simulink model "test_GRM_Airframe"  (R2019b)
settings: Solver=FixedStepAuto  StartTime=0.0  StopTime=60  FixedStep=0.001  RelTol=1e-3
PreLoadFcn:
  | addpath('init_functions');
  | init_grm;
  | addpath('parameters');
  | para_def_grm;
values from neighbouring files (symbols this model uses):
  a_vBEW = 0    [init_grm.m]
  act_dmp = 0.6322    [para_def_grm.m]
  act_omega = 59.9250    (= 59.925)    [para_def_grm.m]
  aero = load('aero.mat')    [para_def_grm.m]
  c_be = -6.5e-3    (= -0.0065)    [init_grm.m]
  c_h_geop0 = 0    [init_grm.m]
  c_h_geope = 11e3    (= 11000)    [init_grm.m]
  c_pa0 = 101325    [init_grm.m]
  c_pe = -c_g0/c_be/sgc    (= 5.25587981272)    [init_grm.m]
  c_r0 = 6371000.79    [init_grm.m]
  c_rot = 7.292115e-5    (= 7.292115e-05)    [init_grm.m]
  c_Tmp0 = 288.15    [init_grm.m]
  chW = pi/2    (= 1.57079632679)    [init_grm.m]
  D = JD - 2451545.0    [init_grm.m]
  d_siB_0 = 0    [para_def_grm.m]
  d_siB_max = deg2rad(1200)    [para_def_grm.m]
  d_siB_min = deg2rad(-1200)    [para_def_grm.m]
  dd_siB_max = deg2rad(50000)    [para_def_grm.m]
  dd_siB_min = deg2rad(-50000)    [para_def_grm.m]
  de_JBBB_xx = JBBB_xx_0 - JBBB_xx_e    (= 0)    [para_def_grm.m]
  de_JBBB_yy = JBBB_yy_0 - JBBB_yy_e    (= 0)    [para_def_grm.m]
  de_JBBB_zz = JBBB_zz_0 - JBBB_zz_e    (= 0)    [para_def_grm.m]
  de_mM = m_fuel_lookup(end)    [para_def_grm.m]
  e_pa = 0    [init_grm.m]
  e_Tmp = 0    [init_grm.m]
  F_prp = [450.52;428.7;423.25;391.61;352.34;304.35;266.17;243.26;216.92 ... (first row only)    [para_def_grm.m]
  flag_I_aero_switch = 1    [init_grm.m]
  flag_I_flat = 1    [init_grm.m]
  flag_I_gravity_switch = 1    [init_grm.m]
  flag_I_rot = 0    [init_grm.m]
  hcr = 1.4    [init_grm.m]
  J0PB_e = TBP*J0PP_e*TBP'    [para_def_grm.m]
  JMMM_0 = TBP*J0PP_0*TBP'    [para_def_grm.m]
  JMMM_e = TBP*J0PP_e*TBP'    [para_def_grm.m]
  lat_0 = 0    [init_grm.m]
  lon_0 = 0    [init_grm.m]
  m0 = mB_0    (= 3.30977)    [para_def_grm.m]
  m_fuel_lookup = [0;0.0573;0.1127;0.1667;0.2186;0.2681;0.3149;0.3588 ... (first row only)    [para_def_grm.m]
  mB_0 = 3.30977    [para_def_grm.m]
  mM_0 = 1.119    [para_def_grm.m]
  mM_e = de_mM    [para_def_grm.m]
  p0PB = [x0PB;y0PB;z0PB]    [para_def_grm.m]
  pBII_0 = TIE_0*pBEE_0    [init_grm.m]
  pMPB = [xMPB;yMPB;zMPB]    [para_def_grm.m]
  pNPB = [0;0;0]    [para_def_grm.m]
  qEG_0 = q12_from_T12(TEG)    [init_grm.m]
  qIB_0 = qumul(qIG_0,qGB_0)    [init_grm.m]
  qIE_0 = q12_from_T12(TIE_0)    [init_grm.m]
  sgc = 287.05287    [init_grm.m]
  siB_0 = 0    [para_def_grm.m]
  siB_max = deg2rad(30)    [para_def_grm.m]
  siB_min = deg2rad(-30)    [para_def_grm.m]
  t_prp1 = [0.04;0.28;0.54;1;1.48;1.99;2.51;3;3.5;3.67;3.82;4]    [para_def_grm.m]
  t_prp2 = t_prp2'    [para_def_grm.m]
  T_sim_lnch = -5    [init_grm.m]
  Tr3r4 = [1,1,1,1;1,1,-1,-1;-1,1,1,-1]*0.25    [para_def_grm.m]
  Tr4r3 = [1,1,-1;1,1,1;1,-1,1;1,-1,-1]    [para_def_grm.m]
  tRRR = 0    [para_def_grm.m]
  unc_a_vBEW_bl = 0    [para_def_grm.m]
  unc_act_bl = 0    [para_def_grm.m]
  unc_act_off = 0    [para_def_grm.m]
  unc_act_scale = 1    [para_def_grm.m]
  unc_aero_Cl_scale = 1    [para_def_grm.m]
  unc_aero_Cm_scale = 1    [para_def_grm.m]
  unc_aero_Cn_scale = 1    [para_def_grm.m]
  unc_aero_Cx_scale = 1    [para_def_grm.m]
  unc_aero_Cy_scale = 1    [para_def_grm.m]
  unc_aero_Cz_scale = 1    [para_def_grm.m]
  unc_cg_x = 0    [para_def_grm.m]
  unc_cg_y = 0    [para_def_grm.m]
  unc_cg_z = 0    [para_def_grm.m]
  unc_chW_bl = 0    [para_def_grm.m]
  unc_fin_def_pitch = 0    [para_def_grm.m]
  unc_fin_def_roll = 0    [para_def_grm.m]
  unc_fin_def_yaw = 0    [para_def_grm.m]
  unc_mB_bl = 0    [para_def_grm.m]
  unc_mB_scale = 1    [para_def_grm.m]
  unc_moi_Jxx = 0    [para_def_grm.m]
  unc_moi_Jyy = 0    [para_def_grm.m]
  unc_moi_Jzz = 0    [para_def_grm.m]
  unc_prp_scale = 1    [para_def_grm.m]
  unc_prp_x = 0    [para_def_grm.m]
  unc_prp_y = 0    [para_def_grm.m]
  unc_prp_z = 0    [para_def_grm.m]
  vBII_0 = vBEE_0 + cross(wIEI_0,pBII_0)    [init_grm.m]
  wBIB_0 = r2_from_r1_trans_q21(wBII_0,qBI_0)    [init_grm.m]
  x0PB = -0.5    [para_def_grm.m]
  xMPB = -0.9    [para_def_grm.m]
  y0PB = 0    [para_def_grm.m]
  yMPB = 0    [para_def_grm.m]
  z0PB = 0    [para_def_grm.m]
  zMPB = 0    [para_def_grm.m]
undefined symbols (not defined in the file or in its folder): c_b_WGS, c_flat, c_grav, c_rsma, d_mB_lookup, t_dmB
libraries: simulink_extras x14, simulink x3
(part 3 of 6)

== system test_GRM_Airframe/GRM_Airframe/rb_eom/calc_bus_flight_dyn_bus_entries/Subsystem2 ==
  TIE : Inport
  pBII : Inport  Port=2
  Constant : Constant  Value=lon_0
  Constant1 : Constant  Value=flag_I_flat
  Constant2 : Constant  Value=lat_0
  Demux : Demux  Outputs=3
  Demux1 : Demux  Outputs=3
  Gain : Gain  Gain=-1
  Math Function : Math  Operator=transpose  SaturateOnIntegerOverflow=on
  Product : Product  Multiplication=Matrix(*)
  Switch : Switch  Criteria=u2 > Threshold
  Terminator : Terminator
  Terminator1 : Terminator
  Vector Concatenate : Concatenate  NumInputs=3
  Vector Concatenate1 : Concatenate  NumInputs=3
  trafo_E_to_geodetic : Subsystem  mask(Transformation der ECEF Position in geodätische Größen){}
      mask help: Dieser Block transformiert die Position im ECEF KOS in die geodätische Länge, Breite und Höhe
      mask init:
      | [c_mue, c_rsma, c_flat] = init_transformations_earth;
      mask Help:
      | Name:
      | 
      |     trafo_E_to_geodetic
      | 
      | Beschreibung:
      | 
      |     Dieser Block transformiert die Position im ECEF KOS in die geodätische
      |     Länge, Breite und Höhe.
      | 
      | Inputs   [size]  [data type] [unit]:
      | 
      |     pBEE    [3] [double] [m]
      | 
      | Outputs  [size]  [data type] [unit]:
      | 
      |     long  [1] [double] [rad]
      |     lat   [1] [double] [rad]
      |     alt   [1] [double] [m]
      | 
      | Parameter
      | 
      |    c_rsma
      |    c_flat
  lon : Outport  VectorParamsAs1DForOutWhenUnconnected=off
  lat : Outport  Port=2  VectorParamsAs1DForOutWhenUnconnected=off
  hBE : Outport  Port=3  VectorParamsAs1DForOutWhenUnconnected=off
  wires:
  Demux1/2 -> lat/1  "lat"
  pBII/1 -> Demux/1, Product/2
  Product/1 -> trafo_E_to_geodetic/1(pBEE)  "pBEE"
  Demux1/1 -> lon/1  "lon"
  Demux1/3 -> hBE/1  "hBE"
  trafo_E_to_geodetic/1(lon) -> Vector Concatenate/1  "lon"
  trafo_E_to_geodetic/2(lat) -> Vector Concatenate/2  "lat"
  trafo_E_to_geodetic/3(alt) -> Vector Concatenate/3  "alt"
  Demux/1 -> Terminator/1
  Demux/2 -> Terminator1/1
  Demux/3 -> Gain/1
  Gain/1 -> Vector Concatenate1/3
  Constant/1 -> Vector Concatenate1/1
  Constant2/1 -> Vector Concatenate1/2
  Vector Concatenate/1 -> Switch/3
  Constant1/1 -> Switch/2
  Vector Concatenate1/1 -> Switch/1
  Switch/1 -> Demux1/1
  TIE/1 -> Math Function/1
  Math Function/1 -> Product/1  "TEI"

== system test_GRM_Airframe/GRM_Airframe/rb_eom/calc_bus_flight_dyn_bus_entries/quaternion_to_euler_angles ==
  note: Inputs [size]:
      |
      | quaternion [4]
  note: Outputs [size]:
      |
      | roll angle [1]
      | pitch angle [1]
      | yaw angle [1]
  note: Um numerische Probleme zu
      | vermeiden, wird hier eine Saturiierung
      | benutzt.
  q : Inport  PortDimensions=4
  Add : Sum
  Add1 : Sum  Inputs=+--
  Add2 : Sum  Inputs=+-
  Add3 : Sum
  Add4 : Sum  Inputs=+--
  Complex to Real-Imag : ComplexToRealImag  Output=Real
  Constant : Constant  Value=0.5
  Constant1 : Constant  Value=0.5
  Demux : Demux
  Gain : Gain  Gain=2
  Product{,1..9} (10 alike) : Product
  Saturation : Saturate  UpperLimit=1  LowerLimit=-1
      settings: AttributesFormatString=|
      | %<UpperLimit>
      | %<LowerLimit>
  Trigonometric Function : Trigonometry  Operator=atan2
  Trigonometric Function1 : Trigonometry  Operator=asin
  Trigonometric Function2 : Trigonometry  Operator=atan2
  Vector Concatenate : Concatenate  NumInputs=3
  eulx : Outport  VectorParamsAs1DForOutWhenUnconnected=off
  wires:
  Saturation/1 -> Trigonometric Function1/1
  Gain/1 -> Saturation/1
  Demux/3 -> Product5/2, Product1/2, Product7/1, Product9/1, Product9/2  "3"
  Constant1/1 -> Add4/1
  Product8/1 -> Add4/2
  Product9/1 -> Add4/3
  Constant/1 -> Add1/1
  Demux/2 -> Product6/2, Product8/1, Product8/2, Product1/1, Product3/1, Product3/2, Product4/1  "2"
  Demux/1 -> Product5/1, Product6/1, Product/1, Product2/1, Product2/2  "1"
  Demux/4 -> Product/2, Product4/2, Product7/2  "4"
  q/1 -> Demux/1
  Add1/1 -> Trigonometric Function/2
  Add2/1 -> Gain/1
  Add4/1 -> Trigonometric Function2/2
  Add3/1 -> Trigonometric Function2/1
  Product6/1 -> Add3/1
  Product7/1 -> Add3/2
  Product4/1 -> Add2/1
  Product5/1 -> Add2/2
  Product2/1 -> Add1/2
  Product3/1 -> Add1/3
  Product/1 -> Add/1
  Product1/1 -> Add/2
  Add/1 -> Trigonometric Function/1
  Trigonometric Function/1 -> Vector Concatenate/1
  Trigonometric Function1/1 -> Vector Concatenate/2
  Trigonometric Function2/1 -> Vector Concatenate/3
  Complex to Real-Imag/1 -> eulx/1
  Vector Concatenate/1 -> Complex to Real-Imag/1

== system test_GRM_Airframe/GRM_Airframe/rb_eom/eom_6dof/Rigid_Body_EOM_6_DOF ==
  FBTX : Inport  PortDimensions=[3,1]
  MBTB : Inport  Port=2  PortDimensions=[3,1]
  mB : Inport  Port=3  PortDimensions=[1]
  x0 : Inport  Port=4
  JBB : Inport  Port=5  PortDimensions=[3,3]
  d_JBB : Inport  Port=6  PortDimensions=[3,3]
  Bus Selector : BusSelector  OutputSignals=qIB,vBII,wBIB
  Constant : Constant  Value=flag_Kraft
  Integration : Subsystem
  Math Function2 : Math  Operator=transpose  SaturateOnIntegerOverflow=on
  Product2 : Product  Multiplication=Matrix(*)
  Switch : Switch  Criteria=u2 > Threshold  Threshold=1
  T12_from_q12 : Subsystem
      mask help: Transforms a quaternion into a Direction Cosine Matrix
      mask Help:
      | Name:
      | 
      |     T12_from_q12
      | 
      | Description:
      | 
      |     This block implements the transformation of a quaternion into the
      |     corresponding direction cosine matrix DCM.
      | 
      | Inputs  [size] [data type] [unit]:
      | 
      |     quaternion q12 [4] [double] [-]
      | 
      | Outputs  [size] [data type] [unit]:
      | 
      |     direction cosine matrix T12  [3x3] [double] [-]
      mask Display:
      | %port_label('input', 1, 'q12')
      | %port_label('output', 1, 'T12')
      | disp('q \rightarrow DCM','texmode','on')
  rb_eom_6dof : Subsystem
  rb_eom : Outport  VectorParamsAs1DForOutWhenUnconnected=off
  wires:
  rb_eom_6dof/4(d_wBIB) -> Integration/4(d_wBIB)  "d_wBIB"
  JBB/1 -> rb_eom_6dof/3(JBB)
  d_JBB/1 -> rb_eom_6dof/5(d_JBB)
  mB/1 -> rb_eom_6dof/2(mB)
  MBTB/1 -> rb_eom_6dof/4(MBTB)
  Switch/1 -> rb_eom_6dof/1(FBTB)
  Constant/1 -> Switch/2
  Product2/1 -> Switch/3
  FBTX/1 -> Product2/2, Switch/1
  Math Function2/1 -> Product2/1
  T12_from_q12/1(T12) -> Math Function2/1
  Bus Selector/2 -> rb_eom_6dof/7(vBII)  "<vBII>"
  x0/1 -> Integration/5(x0)
  Bus Selector/1 -> rb_eom_6dof/6(qIB), T12_from_q12/1(q12)  "<qIB>"
  Bus Selector/3 -> rb_eom_6dof/8(wBIB)  "<wBIB>"
  rb_eom_6dof/1(d_pBII) -> Integration/1(d_pBII)  "d_pBII"
  rb_eom_6dof/2(d_vBII) -> Integration/2(d_vBII)  "d_vBII"
  rb_eom_6dof/3(d_qIB) -> Integration/3(d_qIB)  "d_qIB"
  Integration/1(eom) -> Bus Selector/1, rb_eom/1

== system test_GRM_Airframe/GRM_Airframe/stream_flow/calc_stream_flow/Subsystem1 ==
  vWEB : Inport
  vBEB : Inport  Port=2
  wBIB : Inport  Port=3
  rho : Inport  Port=4
  sos : Inport  Port=5
  AoA_Sideslip_Alphatot_Phi : Subsystem
      mask help:
      | Aus den Komponenten der Geschwindigkeit im ECEF-System, dargestellt im Body-System vBEB
      | werden Anstellwinkel (alpha), Schiebewinkel (beta), totaler Anstellwinkel (alpha_T) sowie Rollwinkel (phi) berechnet.
      | Die Ausgabe erfolgt als Bus in [rad]
      mask Help:
      | Name:
      | 
      |    AoA_sideslip_alphatot_phi
      | 
      | Beschreibung:
      | 
      |   Dieser Block berechnet Anstellwinkel, Schiebewinkel, totalen Anstellwinkel und Rollwinkel in [rad]
      |   aus der Geschwindigkeit vBEB (ECEF-System dargestellt in Body-Koordinaten)
      | 
      | Inputs   [dimension]  [data type] [unit]:
      | 
      |     vBEB    [3] [double] [m/s]
      | 
      | Outputs  [dimension]  [data type] [unit]:
      | 
      | aero_angle_bus [4] [bus] [-]
      |     alpha     [1] [double] [rad]
      |     beta       [1] [double] [rad]
      |     alpha_T [1] [double] [rad]
      |     phi         [1] [double] [rad]
      mask Display:
      | %port_label('input', 1, 'vBEB')
      | %port_label('output', 1, 'aero_angles')
      | disp('vBEB \rightarrow \alpha \beta \alpha_T \phi','texmode','on')
  Bus Selector : BusSelector  OutputSignals=al,be,th,fi
  Constant : Constant  Value=0.5
  Divide : Product  Inputs=*/
  Math Function1 : Math  Operator=square  SaturateOnIntegerOverflow=on
  Product1 : Product  Inputs=3
  Subtract : Sum  Inputs=+-
  calc_nondimensional_rates : Subsystem
  norm_of_vector : Subsystem
      mask help: computes the norm of a vector
      mask Help:
      | Name:
      | 
      |     norm_of_vector
      | 
      | Description:
      | 
      |     This block computes the L2-norm (length) of a vector.
      | 
      | Inputs  [size] [data type] [unit]:
      | 
      |     vector  [3] [double] [-]
      | 
      | Outputs  [size] [data type] [unit]:
      | 
      |     norm of vector  [1] [double] [-]
      mask Display: disp (' norm(r) ')
  al : Outport  VectorParamsAs1DForOutWhenUnconnected=off
  be : Outport  Port=2  VectorParamsAs1DForOutWhenUnconnected=off
  qdynB : Outport  Port=3  VectorParamsAs1DForOutWhenUnconnected=off
  MaB : Outport  Port=4  VectorParamsAs1DForOutWhenUnconnected=off
  a_vB : Outport  Port=5  VectorParamsAs1DForOutWhenUnconnected=off
  wBIB_star : Outport  Port=6  VectorParamsAs1DForOutWhenUnconnected=off
  th : Outport  Port=7  VectorParamsAs1DForOutWhenUnconnected=off
  fi : Outport  Port=8  VectorParamsAs1DForOutWhenUnconnected=off
  wires:
  sos/1 -> Divide/2
  AoA_Sideslip_Alphatot_Phi/1(aero_angles) -> Bus Selector/1
  vBEB/1 -> Subtract/1
  norm_of_vector/1(norm_of_vector) -> Math Function1/1, calc_nondimensional_rates/1(a_vB), a_vB/1, Divide/1  "a_vB"
  Product1/1 -> qdynB/1  "qdynB"
  Math Function1/1 -> Product1/1
  Constant/1 -> Product1/2
  Divide/1 -> MaB/1  "MaB"
  Bus Selector/2 -> be/1  "<be>"
  rho/1 -> Product1/3
  Bus Selector/1 -> al/1  "<al>"
  wBIB/1 -> calc_nondimensional_rates/2(wBIB)
  calc_nondimensional_rates/1(wBIB_star) -> wBIB_star/1
  Bus Selector/3 -> th/1  "<th>"
  Bus Selector/4 -> fi/1  "<fi>"
  vWEB/1 -> Subtract/2
  Subtract/1 -> norm_of_vector/1(vector), AoA_Sideslip_Alphatot_Phi/1(vBEB)  "vBEB_a"

== system test_GRM_Airframe/GRM_Airframe/stream_flow/calc_stream_flow/velocity_vector_transformation ==
  wIEE : Inport
  TIE : Inport  Port=2
  vBII : Inport  Port=3
  pBII : Inport  Port=4
  Add : Sum  Inputs=+-
  Product : Product  Multiplication=Matrix(*)
  cross_product : Subsystem
      mask help: cross product r3 = r1 x r2
      mask Help:
      | Name:
      | 
      |     cross_product
      | 
      | Description:
      | 
      |     This block implements the cross product r3 = r1 x r2.
      | 
      | Inputs  [size] [data type] [unit]:
      | 
      |     vector 1  [3] [double] [-]
      |     vector 2  [3] [double] [-]
      | 
      | Outputs  [size] [data type] [unit]:
      | 
      |     resulting vector  [3] [double] [-]
      mask Display: disp(' r3 = r1 x r2')
  vBEI : Outport  VectorParamsAs1DForOutWhenUnconnected=off
  wires:
  TIE/1 -> Product/1
  wIEE/1 -> Product/2
  Product/1 -> cross_product/1(r1)  "wIEI"
  pBII/1 -> cross_product/2(r2)
  cross_product/1(r1_x_r2) -> Add/2  "de_vBEI"
  vBII/1 -> Add/1
  Add/1 -> vBEI/1  "vBEI"

== system test_GRM_Airframe/GRM_Airframe/weight_and_balance/d_moi/vector2diagonal_matrix ==
  vector : Inport
  Constant6 : Constant  Value=0
  Demux : Demux  Outputs=3
  Vector Concatenate1 : Concatenate  NumInputs=3
  Vector Concatenate2 : Concatenate  NumInputs=3
  Vector Concatenate3 : Concatenate  NumInputs=3
  Vector Concatenate4 : Concatenate  NumInputs=3  Mode=Multidimensional array  ConcatenateDimension=2
  diagonal_matrix : Outport  VectorParamsAs1DForOutWhenUnconnected=off
  wires:
  Demux/1 -> Vector Concatenate1/1
  vector/1 -> Demux/1
  Constant6/1 -> Vector Concatenate3/2, Vector Concatenate3/1, Vector Concatenate2/3, Vector Concatenate2/1, Vector Concatenate1/3, Vector Concatenate1/2
  Vector Concatenate4/1 -> diagonal_matrix/1
  Demux/2 -> Vector Concatenate2/2
  Vector Concatenate2/1 -> Vector Concatenate4/2
  Vector Concatenate1/1 -> Vector Concatenate4/1
  Vector Concatenate3/1 -> Vector Concatenate4/3
  Demux/3 -> Vector Concatenate3/3

== system test_GRM_Airframe/GRM_Airframe/weight_and_balance/moi/JMMM_linear_interpolation ==
  mM : Inport
  Constant16 : Constant  Value=JMMM_0
  Constant17 : Constant  Value=JMMM_e
  Constant18 : Constant  Value=mM_0
  Constant19 : Constant  Value=mM_e
  Constant20 : Constant  Value=mM_0
  Constant21 : Constant  Value=JMMM_0
  Divide : Product  Inputs=**/
  Subtract : Sum  Inputs=+-
  Subtract4 : Sum  Inputs=+-
  Subtract5 : Sum  Inputs=+-
  Subtract6 : Sum
  JMMM : Outport  VectorParamsAs1DForOutWhenUnconnected=off
  wires:
  mM/1 -> Subtract5/1
  Subtract5/1 -> Divide/1
  Constant20/1 -> Subtract5/2
  Constant19/1 -> Subtract4/1
  Constant18/1 -> Subtract4/2
  Constant17/1 -> Subtract/1
  Constant16/1 -> Subtract/2
  Subtract/1 -> Divide/2
  Subtract4/1 -> Divide/3
  Subtract6/1 -> JMMM/1  "JMMM"
  Constant21/1 -> Subtract6/1
  Divide/1 -> Subtract6/2

== system test_GRM_Airframe/GRM_Airframe/weight_and_balance/moi/moi_coordinate_transformation ==
  JMMM : Inport
  3_rot_mat : Subsystem  mask(Rotation um 1, 2 oder 3 Achsen){rot_1=Rotation um z-Achse, rot_2=Rotation um y-Achse, rot_3=Rotation um x-Achse}
      mask prompts: rot_1 "1. Rotation"; rot_2 "2. Rotation"; rot_3 "3. Rotation"
      mask help:
      | Dieser Block liefert die Rotationsmatrix T12 für den Fall zurück, dass sich das Ziel-Koordinatensystem (1) durch Drehungen um 1, 2 oder 3 Achsen gegenüber dem Ausgangskoordinatensystem (2) beschreiben lässt (passive Drehung).
      |
      | Die Anzahl der Rotation sowie die Reihenfolge ist frei einstellbar.
      |
      | Die Rotationswinkel haben die Einheit [rad].
      mask TypeOptions rot_1: Rotation um x-Achse | Rotation um y-Achse | Rotation um z-Achse
      mask TypeOptions rot_2: Rotation um x-Achse | Rotation um y-Achse | Rotation um z-Achse
      mask TypeOptions rot_3: Rotation um x-Achse | Rotation um y-Achse | Rotation um z-Achse
  Math Function : Math  Operator=transpose  SaturateOnIntegerOverflow=on
  Matrix Multiply : Product  Multiplication=Matrix(*)
  Matrix Multiply1 : Product  Multiplication=Matrix(*)
  Thrust_rot_z : Constant  Value=unc_prp_z
  thrust_rot_x : Constant  Value=unc_prp_x
  thrust_rot_y : Constant  Value=unc_prp_y
  JMMB : Outport  VectorParamsAs1DForOutWhenUnconnected=off
  wires:
  Math Function/1 -> Matrix Multiply1/2
  Matrix Multiply/1 -> Matrix Multiply1/1
  JMMM/1 -> Matrix Multiply/2
  3_rot_mat/1(T12) -> Math Function/1, Matrix Multiply/1
  Matrix Multiply1/1 -> JMMB/1  "JMMB"
  thrust_rot_y/1 -> 3_rot_mat/2(wi2)
  thrust_rot_x/1 -> 3_rot_mat/3(wi3)
  Thrust_rot_z/1 -> 3_rot_mat/1(wi1)

== system test_GRM_Airframe/GRM_Airframe/weight_and_balance/moi/moi_uncertainty ==
  JBBB_c : Inport
  Add7 : Sum
  Constant16 : Constant  Value=[unc_moi_Jxx,0,0;0,unc_moi_Jyy,0;0,0,unc_moi_Jzz]
  JBBB : Outport  VectorParamsAs1DForOutWhenUnconnected=off
  wires:
  Add7/1 -> JBBB/1  "JBBB"
  JBBB_c/1 -> Add7/1
  Constant16/1 -> Add7/2

== system test_GRM_Airframe/GRM_Airframe/weight_and_balance/moi/steiners_theorem_missile ==
  pBPB : Inport
  Constant : Constant  Value=mB_0
  Constant17 : Constant  Value=p0PB
  Product : Product
  Subtract : Sum  Inputs=+-
  create_deviation_matrix : Subsystem
  J_deviation : Outport  VectorParamsAs1DForOutWhenUnconnected=off
  wires:
  pBPB/1 -> Subtract/1
  Product/1 -> J_deviation/1
  create_deviation_matrix/1(T_deviation) -> Product/2
  Constant17/1 -> Subtract/2
  Subtract/1 -> create_deviation_matrix/1(pBXB)  "pB0B"
  Constant/1 -> Product/1

== system test_GRM_Airframe/GRM_Airframe/weight_and_balance/moi/steiners_theorem_motor ==
  pBPB : Inport
  mM : Inport  Port=2
  Constant16 : Constant  Value=pMPB
  Product : Product
  Subtract4 : Sum  Inputs=+-
  create_deviation_matrix1 : Subsystem
  JM_deviation : Outport  VectorParamsAs1DForOutWhenUnconnected=off
  wires:
  Product/1 -> JM_deviation/1
  pBPB/1 -> Subtract4/1
  create_deviation_matrix1/1(T_deviation) -> Product/1
  Constant16/1 -> Subtract4/2
  Subtract4/1 -> create_deviation_matrix1/1(pBXB)  "pBMB"
  mM/1 -> Product/2

== system test_GRM_Airframe/environment_global/weather/atm_dynamic/trafo_around_z_axis ==
  vec1 : Inport
  gamma : Inport  Port=2
  1_rot_mat : Subsystem  mask(Rotation um 1, 2 oder 3 Achsen){rot_1=Rotation um z-Achse}
      mask prompts: rot_1 "1. Rotation"
      mask help:
      | Dieser Block liefert die Rotationsmatrix T12 für den Fall zurück, dass sich das Ziel-Koordinatensystem (1) durch Drehungen um 1, 2 oder 3 Achsen gegenüber dem Ausgangskoordinatensystem (2) beschreiben lässt (passive Drehung).
      |
      | Die Anzahl der Rotation sowie die Reihenfolge ist frei einstellbar.
      |
      | Die Rotationswinkel haben die Einheit [rad].
      mask TypeOptions rot_1: Rotation um x-Achse | Rotation um y-Achse | Rotation um z-Achse
  Product : Product  Multiplication=Matrix(*)
  Reshape : Reshape  OutputDimensionality=Column vector (2-D)
  vec2 : Outport  VectorParamsAs1DForOutWhenUnconnected=off
  wires:
  Reshape/1 -> Product/2  "vec1"
  vec1/1 -> Reshape/1  "vec1"
  1_rot_mat/1(T12) -> Product/1  "T12"
  gamma/1 -> 1_rot_mat/1(wi1)  "gamma"
  Product/1 -> vec2/1  "vec2"

== system test_GRM_Airframe/GRM_Airframe/aerodynamics/aerodynamic_via_lookup/calc_aero_for_mom/cross_product ==
  note: Outputs [size]:
      |
      | r1 x r2  [3x1]
  note: Inputs [size]:
      |
      | r1 [3x1]
      | r2 [3x1]
  r1 : Inport
  r2 : Inport  Port=2
  Demux2 : Demux  Outputs=[1;1;1]
  Demux3 : Demux  Outputs=[1;1;1]
  Product{2..7} (6 alike) : Product  SaturateOnIntegerOverflow=on  RndMeth=Zero  InputSameDT=on  OutDataTypeStr=Inherit: Same as first input
  Sum : Sum  Inputs=+-  SaturateOnIntegerOverflow=on  InputSameDT=on  OutDataTypeStr=Inherit: Same as first input
  Sum1 : Sum  Inputs=+-  SaturateOnIntegerOverflow=on  InputSameDT=on  OutDataTypeStr=Inherit: Same as first input
  Sum2 : Sum  Inputs=+-  SaturateOnIntegerOverflow=on  InputSameDT=on  OutDataTypeStr=Inherit: Same as first input
  Vector Concatenate : Concatenate  NumInputs=3  Mode=Multidimensional array
  r1_x_r2 : Outport  PortDimensions=[3,1]  VectorParamsAs1DForOutWhenUnconnected=off
  wires:
  Demux2/2 -> Product2/1, Product7/1
  Demux3/3 -> Product5/2, Product2/2
  Demux3/2 -> Product6/2, Product3/2
  Demux2/3 -> Product3/1, Product4/1
  Demux3/1 -> Product7/2, Product4/2
  Demux2/1 -> Product6/1, Product5/1
  Product2/1 -> Sum/1
  Product3/1 -> Sum/2
  Product4/1 -> Sum1/1
  Product5/1 -> Sum1/2
  Product6/1 -> Sum2/1
  Product7/1 -> Sum2/2
  Sum/1 -> Vector Concatenate/1
  Sum1/1 -> Vector Concatenate/2
  Sum2/1 -> Vector Concatenate/3
  r1/1 -> Demux2/1
  r2/1 -> Demux3/1
  Vector Concatenate/1 -> r1_x_r2/1

== system test_GRM_Airframe/GRM_Airframe/aerodynamics/aerodynamic_via_lookup/calc_aero_for_mom/launch_rail ==
  hBE : Inport
  FBAB_c : Inport  Port=2
  Constant1 : Constant  Value=flag_I_aero_switch
  Constant3 : Constant  Value=0
  Subtract : Sum  Inputs=++-
  Switch : Switch  Criteria=u2 > Threshold  Threshold=0.05
  Vector Concatenate : Concatenate  NumInputs=3
  initial_altitude : Subsystem
  FBAB : Outport  VectorParamsAs1DForOutWhenUnconnected=off
  wires:
  Constant1/1 -> Subtract/2
  hBE/1 -> Subtract/1
  Subtract/1 -> Switch/2
  Constant3/1 -> Vector Concatenate/1, Vector Concatenate/2, Vector Concatenate/3
  Switch/1 -> FBAB/1  "FBAB"
  Vector Concatenate/1 -> Switch/3
  FBAB_c/1 -> Switch/1
  initial_altitude/1(hBE_0) -> Subtract/3

== system test_GRM_Airframe/GRM_Airframe/aerodynamics/aerodynamic_via_lookup/calc_aero_for_mom/launch_rail1 ==
  hBE : Inport
  MBAB_c : Inport  Port=2
  Constant1 : Constant  Value=flag_I_aero_switch
  Constant3 : Constant  Value=0
  Subtract : Sum  Inputs=++-
  Switch : Switch  Criteria=u2 > Threshold  Threshold=0.05
  Vector Concatenate : Concatenate  NumInputs=3
  initial_altitude : Subsystem
  MBAB : Outport  VectorParamsAs1DForOutWhenUnconnected=off
  wires:
  initial_altitude/1(hBE_0) -> Subtract/3
  MBAB_c/1 -> Switch/1
  Vector Concatenate/1 -> Switch/3
  Switch/1 -> MBAB/1  "MBAB"
  Constant3/1 -> Vector Concatenate/3, Vector Concatenate/2, Vector Concatenate/1
  Subtract/1 -> Switch/2
  hBE/1 -> Subtract/1
  Constant1/1 -> Subtract/2

== system test_GRM_Airframe/GRM_Airframe/aerodynamics/aerodynamic_via_lookup/calc_derivatives/Cl_derivatives_lookup ==
  aero_pre_lookup : Inport
  Bus Creator1 : BusCreator  Inputs=7
  Bus Selector2 : BusSelector  OutputSignals=k_Mach,f_Mach,k_alB,f_alB,k_beB,f_beB
  Cl_Interpolation : Interpolation_n-D  NumberOfTableDimensions=3  Table=aero.Cl  ExtrapMethod=Clip  DiagnosticForOutOfRangeInput=Warning  InternalRulePriority=Speed
      settings: InputPortMap=u0,u1,u2,u3,u4,u5
  Cl_delta_l_Interpolation : Interpolation_n-D  NumberOfTableDimensions=3  Table=aero.Cl_delta_l  ExtrapMethod=Clip  DiagnosticForOutOfRangeInput=Warning  InternalRulePriority=Speed
      settings: InputPortMap=u0,u1,u2,u3,u4,u5
  Cl_delta_m_Interpolation : Interpolation_n-D  NumberOfTableDimensions=3  Table=aero.Cl_delta_m  ExtrapMethod=Clip  DiagnosticForOutOfRangeInput=Warning  InternalRulePriority=Speed
      settings: InputPortMap=u0,u1,u2,u3,u4,u5
  Cl_delta_n_Interpolation : Interpolation_n-D  NumberOfTableDimensions=3  Table=aero.Cl_delta_n  ExtrapMethod=Clip  DiagnosticForOutOfRangeInput=Warning  InternalRulePriority=Speed
      settings: InputPortMap=u0,u1,u2,u3,u4,u5
  Clp_Interpolation : Interpolation_n-D  NumberOfTableDimensions=3  Table=aero.Clp  ExtrapMethod=Clip  DiagnosticForOutOfRangeInput=Warning  InternalRulePriority=Speed
      settings: InputPortMap=u0,u1,u2,u3,u4,u5
  Clq_Interpolation : Interpolation_n-D  NumberOfTableDimensions=3  Table=aero.Clq  ExtrapMethod=Clip  DiagnosticForOutOfRangeInput=Warning  InternalRulePriority=Speed
      settings: InputPortMap=u0,u1,u2,u3,u4,u5
  Clr_Interpolation : Interpolation_n-D  NumberOfTableDimensions=3  Table=aero.Clr  ExtrapMethod=Clip  DiagnosticForOutOfRangeInput=Warning  InternalRulePriority=Speed
      settings: InputPortMap=u0,u1,u2,u3,u4,u5
  Constant : Constant  Value=unc_aero_Cl_scale
  Product : Product
  Cl_deriv : Outport  VectorParamsAs1DForOutWhenUnconnected=off
  wires:
  Bus Selector2/6 -> Cl_delta_n_Interpolation/6, Cl_delta_m_Interpolation/6, Cl_delta_l_Interpolation/6, Clr_Interpolation/6, Clq_Interpolation/6, Clp_Interpolation/6, Cl_Interpolation/6  "<f_beB>"
  Bus Selector2/4 -> Cl_delta_n_Interpolation/4, Cl_delta_m_Interpolation/4, Cl_delta_l_Interpolation/4, Clr_Interpolation/4, Clq_Interpolation/4, Clp_Interpolation/4, Cl_Interpolation/4  "<f_alB>"
  Bus Selector2/3 -> Cl_delta_n_Interpolation/3, Cl_delta_m_Interpolation/3, Cl_delta_l_Interpolation/3, Clr_Interpolation/3, Clq_Interpolation/3, Clp_Interpolation/3, Cl_Interpolation/3  "<k_alB>"
  Bus Selector2/2 -> Cl_delta_n_Interpolation/2, Cl_delta_m_Interpolation/2, Cl_delta_l_Interpolation/2, Clr_Interpolation/2, Clq_Interpolation/2, Clp_Interpolation/2, Cl_Interpolation/2  "<f_Mach>"
  Bus Selector2/1 -> Cl_delta_n_Interpolation/1, Cl_delta_m_Interpolation/1, Cl_delta_l_Interpolation/1, Clr_Interpolation/1, Clq_Interpolation/1, Clp_Interpolation/1, Cl_Interpolation/1  "<k_Mach>"
  Bus Selector2/5 -> Cl_delta_n_Interpolation/5, Cl_delta_m_Interpolation/5, Cl_delta_l_Interpolation/5, Clr_Interpolation/5, Clq_Interpolation/5, Clp_Interpolation/5, Cl_Interpolation/5  "<k_beB>"
  Cl_delta_n_Interpolation/1 -> Bus Creator1/7  "Cldn"
  Clq_Interpolation/1 -> Bus Creator1/3  "Clq"
  Clr_Interpolation/1 -> Bus Creator1/4  "Clr"
  Cl_delta_m_Interpolation/1 -> Bus Creator1/6  "Cldm"
  Cl_Interpolation/1 -> Product/2  "Cl"
  aero_pre_lookup/1 -> Bus Selector2/1
  Cl_delta_l_Interpolation/1 -> Bus Creator1/5  "Cldl"
  Clp_Interpolation/1 -> Bus Creator1/2  "Clp"
  Bus Creator1/1 -> Cl_deriv/1  "Cl_deriv_bus"
  Constant/1 -> Product/1
  Product/1 -> Bus Creator1/1  "Cl"

== system test_GRM_Airframe/GRM_Airframe/aerodynamics/aerodynamic_via_lookup/calc_derivatives/Cm_derivatives_lookup ==
  aero_pre_lookup : Inport
  Bus Creator1 : BusCreator  Inputs=7
  Bus Selector2 : BusSelector  OutputSignals=k_Mach,f_Mach,k_alB,f_alB,k_beB,f_beB
  Cm_Interpolation : Interpolation_n-D  NumberOfTableDimensions=3  Table=aero.Cm  ExtrapMethod=Clip  DiagnosticForOutOfRangeInput=Warning  InternalRulePriority=Speed
      settings: InputPortMap=u0,u1,u2,u3,u4,u5
  Cm_delta_l_Interpolation : Interpolation_n-D  NumberOfTableDimensions=3  Table=aero.Cm_delta_l  ExtrapMethod=Clip  DiagnosticForOutOfRangeInput=Warning  InternalRulePriority=Speed
      settings: InputPortMap=u0,u1,u2,u3,u4,u5
  Cm_delta_m_Interpolation : Interpolation_n-D  NumberOfTableDimensions=3  Table=aero.Cm_delta_m  ExtrapMethod=Clip  DiagnosticForOutOfRangeInput=Warning  InternalRulePriority=Speed
      settings: InputPortMap=u0,u1,u2,u3,u4,u5
  Cm_delta_n_Interpolation : Interpolation_n-D  NumberOfTableDimensions=3  Table=aero.Cm_delta_n  ExtrapMethod=Clip  DiagnosticForOutOfRangeInput=Warning  InternalRulePriority=Speed
      settings: InputPortMap=u0,u1,u2,u3,u4,u5
  Cmp_Interpolation : Interpolation_n-D  NumberOfTableDimensions=3  Table=aero.Cmp  ExtrapMethod=Clip  DiagnosticForOutOfRangeInput=Warning  InternalRulePriority=Speed
      settings: InputPortMap=u0,u1,u2,u3,u4,u5
  Cmq_Interpolation : Interpolation_n-D  NumberOfTableDimensions=3  Table=aero.Cmq  ExtrapMethod=Clip  DiagnosticForOutOfRangeInput=Warning  InternalRulePriority=Speed
      settings: InputPortMap=u0,u1,u2,u3,u4,u5
  Cmr_Interpolation : Interpolation_n-D  NumberOfTableDimensions=3  Table=aero.Cmr  ExtrapMethod=Clip  DiagnosticForOutOfRangeInput=Warning  InternalRulePriority=Speed
      settings: InputPortMap=u0,u1,u2,u3,u4,u5
  Constant : Constant  Value=unc_aero_Cm_scale
  Product : Product
  Cm_deriv : Outport  VectorParamsAs1DForOutWhenUnconnected=off
  wires:
  Bus Creator1/1 -> Cm_deriv/1  "Cm_deriv_bus"
  Cmr_Interpolation/1 -> Bus Creator1/4  "Cmr"
  Cm_delta_m_Interpolation/1 -> Bus Creator1/6  "Cmdm"
  Cm_delta_n_Interpolation/1 -> Bus Creator1/7  "Cmdn"
  Cm_Interpolation/1 -> Product/2  "Cm"
  Cmq_Interpolation/1 -> Bus Creator1/3  "Cmq"
  Bus Selector2/5 -> Cm_delta_n_Interpolation/5, Cm_delta_m_Interpolation/5, Cm_delta_l_Interpolation/5, Cmr_Interpolation/5, Cmq_Interpolation/5, Cmp_Interpolation/5, Cm_Interpolation/5  "<k_beB>"
  Cm_delta_l_Interpolation/1 -> Bus Creator1/5  "Cmdl"
  Cmp_Interpolation/1 -> Bus Creator1/2  "Cmp"
  aero_pre_lookup/1 -> Bus Selector2/1
  Bus Selector2/6 -> Cm_delta_n_Interpolation/6, Cm_delta_m_Interpolation/6, Cm_delta_l_Interpolation/6, Cmr_Interpolation/6, Cmq_Interpolation/6, Cmp_Interpolation/6, Cm_Interpolation/6  "<f_beB>"
  Bus Selector2/1 -> Cm_delta_n_Interpolation/1, Cm_delta_m_Interpolation/1, Cm_delta_l_Interpolation/1, Cmr_Interpolation/1, Cmq_Interpolation/1, Cmp_Interpolation/1, Cm_Interpolation/1  "<k_Mach>"
  Bus Selector2/2 -> Cm_delta_n_Interpolation/2, Cm_delta_m_Interpolation/2, Cm_delta_l_Interpolation/2, Cmr_Interpolation/2, Cmq_Interpolation/2, Cmp_Interpolation/2, Cm_Interpolation/2  "<f_Mach>"
  Bus Selector2/3 -> Cm_delta_n_Interpolation/3, Cm_delta_m_Interpolation/3, Cm_delta_l_Interpolation/3, Cmr_Interpolation/3, Cmq_Interpolation/3, Cmp_Interpolation/3, Cm_Interpolation/3  "<k_alB>"
  Bus Selector2/4 -> Cm_delta_n_Interpolation/4, Cm_delta_m_Interpolation/4, Cm_delta_l_Interpolation/4, Cmr_Interpolation/4, Cmq_Interpolation/4, Cmp_Interpolation/4, Cm_Interpolation/4  "<f_alB>"
  Constant/1 -> Product/1
  Product/1 -> Bus Creator1/1  "Cm"

== system test_GRM_Airframe/GRM_Airframe/aerodynamics/aerodynamic_via_lookup/calc_derivatives/Cn_derivatives_lookup ==
  aero_pre_lookup : Inport
  Bus Creator1 : BusCreator  Inputs=7
  Bus Selector1 : BusSelector  OutputSignals=k_Mach,f_Mach,k_alB,f_alB,k_beB,f_beB
  Cn_Interpolation : Interpolation_n-D  NumberOfTableDimensions=3  Table=aero.Cn  ExtrapMethod=Clip  DiagnosticForOutOfRangeInput=Warning  InternalRulePriority=Speed
      settings: InputPortMap=u0,u1,u2,u3,u4,u5
  Cn_delta_l_Interpolation : Interpolation_n-D  NumberOfTableDimensions=3  Table=aero.Cn_delta_l  ExtrapMethod=Clip  DiagnosticForOutOfRangeInput=Warning  InternalRulePriority=Speed
      settings: InputPortMap=u0,u1,u2,u3,u4,u5
  Cn_delta_m_Interpolation : Interpolation_n-D  NumberOfTableDimensions=3  Table=aero.Cn_delta_m  ExtrapMethod=Clip  DiagnosticForOutOfRangeInput=Warning  InternalRulePriority=Speed
      settings: InputPortMap=u0,u1,u2,u3,u4,u5
  Cn_delta_n_Interpolation : Interpolation_n-D  NumberOfTableDimensions=3  Table=aero.Cn_delta_n  ExtrapMethod=Clip  DiagnosticForOutOfRangeInput=Warning  InternalRulePriority=Speed
      settings: InputPortMap=u0,u1,u2,u3,u4,u5
  Cnp_Interpolation : Interpolation_n-D  NumberOfTableDimensions=3  Table=aero.Cnp  ExtrapMethod=Clip  DiagnosticForOutOfRangeInput=Warning  InternalRulePriority=Speed
      settings: InputPortMap=u0,u1,u2,u3,u4,u5
  Cnq_Interpolation : Interpolation_n-D  NumberOfTableDimensions=3  Table=aero.Cnq  ExtrapMethod=Clip  DiagnosticForOutOfRangeInput=Warning  InternalRulePriority=Speed
      settings: InputPortMap=u0,u1,u2,u3,u4,u5
  Cnr_Interpolation : Interpolation_n-D  NumberOfTableDimensions=3  Table=aero.Cnr  ExtrapMethod=Clip  DiagnosticForOutOfRangeInput=Warning  InternalRulePriority=Speed
      settings: InputPortMap=u0,u1,u2,u3,u4,u5
  Constant : Constant  Value=unc_aero_Cn_scale
  Product : Product
  Cn_deriv : Outport  VectorParamsAs1DForOutWhenUnconnected=off
  wires:
  Bus Selector1/3 -> Cn_delta_n_Interpolation/3, Cn_delta_m_Interpolation/3, Cn_delta_l_Interpolation/3, Cnr_Interpolation/3, Cnq_Interpolation/3, Cnp_Interpolation/3, Cn_Interpolation/3  "<k_alB>"
  Bus Selector1/4 -> Cn_delta_n_Interpolation/4, Cn_delta_m_Interpolation/4, Cn_delta_l_Interpolation/4, Cnr_Interpolation/4, Cnq_Interpolation/4, Cnp_Interpolation/4, Cn_Interpolation/4  "<f_alB>"
  Bus Selector1/1 -> Cn_delta_n_Interpolation/1, Cn_delta_m_Interpolation/1, Cn_delta_l_Interpolation/1, Cnr_Interpolation/1, Cnq_Interpolation/1, Cnp_Interpolation/1, Cn_Interpolation/1  "<k_Mach>"
  Bus Selector1/2 -> Cn_delta_n_Interpolation/2, Cn_delta_m_Interpolation/2, Cn_delta_l_Interpolation/2, Cnr_Interpolation/2, Cnq_Interpolation/2, Cnp_Interpolation/2, Cn_Interpolation/2  "<f_Mach>"
  aero_pre_lookup/1 -> Bus Selector1/1
  Cnp_Interpolation/1 -> Bus Creator1/2  "Cnp"
  Bus Creator1/1 -> Cn_deriv/1  "Cn_deriv_bus"
  Bus Selector1/5 -> Cn_delta_n_Interpolation/5, Cn_delta_m_Interpolation/5, Cn_delta_l_Interpolation/5, Cnr_Interpolation/5, Cnq_Interpolation/5, Cnp_Interpolation/5, Cn_Interpolation/5  "<k_beB>"
  Cnr_Interpolation/1 -> Bus Creator1/4  "Cnr"
  Cnq_Interpolation/1 -> Bus Creator1/3  "Cnq"
  Cn_delta_m_Interpolation/1 -> Bus Creator1/6  "Cndm"
  Cn_Interpolation/1 -> Product/2  "Cn"
  Cn_delta_n_Interpolation/1 -> Bus Creator1/7  "Cndn"
  Cn_delta_l_Interpolation/1 -> Bus Creator1/5  "Cndl"
  Bus Selector1/6 -> Cn_delta_n_Interpolation/6, Cn_delta_m_Interpolation/6, Cn_delta_l_Interpolation/6, Cnr_Interpolation/6, Cnq_Interpolation/6, Cnp_Interpolation/6, Cn_Interpolation/6  "<f_beB>"
  Constant/1 -> Product/1
  Product/1 -> Bus Creator1/1  "Cn"

== system test_GRM_Airframe/GRM_Airframe/aerodynamics/aerodynamic_via_lookup/calc_derivatives/Cx_derivatives_lookup ==
  delta_t : Inport
  hBE : Inport  Port=2
  aero_pre_lookup : Inport  Port=3
  Bus Creator1 : BusCreator  Inputs=10
  Bus Selector1 : BusSelector  OutputSignals=k_Mach,f_Mach,k_alB,f_alB,k_beB,f_beB
  Constant : Constant  Value=unc_aero_Cx_scale
  Cx_Interpolation : Interpolation_n-D  NumberOfTableDimensions=3  Table=aero.Cx  ExtrapMethod=Clip  InternalRulePriority=Speed
      settings: InputPortMap=u0,u1,u2,u3,u4,u5
  Cx_alt_Interpolation : Interpolation_n-D  NumberOfTableDimensions=3  Table=aero.Cx_alt  ExtrapMethod=Clip  InternalRulePriority=Speed
      settings: InputPortMap=u0,u1,u2,u3,u4,u5
  Cx_base_Interpolation : Interpolation_n-D  NumberOfTableDimensions=3  Table=aero.Cx_base  ExtrapMethod=Clip  InternalRulePriority=Speed
      settings: InputPortMap=u0,u1,u2,u3,u4,u5
  Cx_delta_l_Interpolation : Interpolation_n-D  NumberOfTableDimensions=3  Table=aero.Cx_delta_l  ExtrapMethod=Clip  InternalRulePriority=Speed
      settings: InputPortMap=u0,u1,u2,u3,u4,u5
  Cx_delta_m_Interpolation : Interpolation_n-D  NumberOfTableDimensions=3  Table=aero.Cx_delta_m  ExtrapMethod=Clip  InternalRulePriority=Speed
      settings: InputPortMap=u0,u1,u2,u3,u4,u5
  Cx_delta_n_Interpolation : Interpolation_n-D  NumberOfTableDimensions=3  Table=aero.Cx_delta_n  ExtrapMethod=Clip  InternalRulePriority=Speed
      settings: InputPortMap=u0,u1,u2,u3,u4,u5
  Cx_delta_t_Interpolation : Interpolation_n-D  NumberOfTableDimensions=3  Table=aero.Cx_delta_t  ExtrapMethod=Clip  InternalRulePriority=Speed
      settings: InputPortMap=u0,u1,u2,u3,u4,u5
  Cxp_Interpolation : Interpolation_n-D  NumberOfTableDimensions=3  Table=aero.Cxp  ExtrapMethod=Clip  InternalRulePriority=Speed
      settings: InputPortMap=u0,u1,u2,u3,u4,u5
  Cxq_Interpolation : Interpolation_n-D  NumberOfTableDimensions=3  Table=aero.Cxq  ExtrapMethod=Clip  InternalRulePriority=Speed
      settings: InputPortMap=u0,u1,u2,u3,u4,u5
  Cxr_Interpolation : Interpolation_n-D  NumberOfTableDimensions=3  Table=aero.Cxr  ExtrapMethod=Clip  InternalRulePriority=Speed
      settings: InputPortMap=u0,u1,u2,u3,u4,u5
  Prelookup_altitude : PreLookup  BreakpointsData=aero.hoehe
  Prelookup_delta_t : PreLookup  BreakpointsData=aero.delta_t
  Product : Product
  Cx_deriv : Outport  VectorParamsAs1DForOutWhenUnconnected=off
  wires:
  Bus Selector1/5 -> Cx_Interpolation/5, Cx_delta_m_Interpolation/5, Cx_delta_n_Interpolation/5, Cx_base_Interpolation/5, Cx_delta_l_Interpolation/5, Cxr_Interpolation/5, Cxq_Interpolation/5, Cxp_Interpolation/5  "<k_beB>"
  Cx_alt_Interpolation/1 -> Bus Creator1/9  "Cx_alt"
  Cx_Interpolation/1 -> Product/2  "Cx"
  Cx_base_Interpolation/1 -> Bus Creator1/8  "Cx_base"
  Cxq_Interpolation/1 -> Bus Creator1/3  "Cxq"
  Cxr_Interpolation/1 -> Bus Creator1/4  "Cxr"
  Cx_delta_t_Interpolation/1 -> Bus Creator1/10  "Cx_alB_t"
  Cxp_Interpolation/1 -> Bus Creator1/2  "Cxp"
  Bus Selector1/4 -> Cx_delta_m_Interpolation/4, Cx_delta_n_Interpolation/4, Cx_base_Interpolation/4, Cx_delta_t_Interpolation/4, Cx_alt_Interpolation/4, Cx_delta_l_Interpolation/4, Cxr_Interpolation/4, Cxq_Interpolation/4, Cxp_Interpolation/4, Cx_Interpolation/4  "<f_alB>"
  Bus Selector1/6 -> Cx_Interpolation/6, Cx_delta_m_Interpolation/6, Cx_delta_n_Interpolation/6, Cx_base_Interpolation/6, Cx_delta_l_Interpolation/6, Cxr_Interpolation/6, Cxq_Interpolation/6, Cxp_Interpolation/6  "<f_beB>"
  Bus Selector1/3 -> Cx_delta_m_Interpolation/3, Cx_delta_n_Interpolation/3, Cx_base_Interpolation/3, Cx_delta_t_Interpolation/3, Cx_alt_Interpolation/3, Cx_delta_l_Interpolation/3, Cxr_Interpolation/3, Cxq_Interpolation/3, Cxp_Interpolation/3, Cx_Interpolation/3  "<k_alB>"
  Prelookup_delta_t/2 -> Cx_delta_t_Interpolation/6
  Bus Selector1/2 -> Cx_delta_m_Interpolation/2, Cx_delta_n_Interpolation/2, Cx_delta_t_Interpolation/2, Cx_alt_Interpolation/2, Cx_base_Interpolation/2, Cx_delta_l_Interpolation/2, Cxr_Interpolation/2, Cxq_Interpolation/2, Cxp_Interpolation/2, Cx_Interpolation/2  "<f_Mach>"
  Bus Selector1/1 -> Cx_delta_m_Interpolation/1, Cx_delta_n_Interpolation/1, Cx_base_Interpolation/1, Cx_delta_t_Interpolation/1, Cx_alt_Interpolation/1, Cx_delta_l_Interpolation/1, Cxr_Interpolation/1, Cxq_Interpolation/1, Cxp_Interpolation/1, Cx_Interpolation/1  "<k_Mach>"
  Prelookup_delta_t/1 -> Cx_delta_t_Interpolation/5
  aero_pre_lookup/1 -> Bus Selector1/1
  hBE/1 -> Prelookup_altitude/1
  Prelookup_altitude/1 -> Cx_alt_Interpolation/5
  Prelookup_altitude/2 -> Cx_alt_Interpolation/6
  Bus Creator1/1 -> Cx_deriv/1  "Cx_deriv_bus"
  delta_t/1 -> Prelookup_delta_t/1
  Cx_delta_l_Interpolation/1 -> Bus Creator1/5  "Cxdl"
  Cx_delta_m_Interpolation/1 -> Bus Creator1/6  "Cxdm"
  Cx_delta_n_Interpolation/1 -> Bus Creator1/7  "Cxdn"
  Product/1 -> Bus Creator1/1  "Cx"
  Constant/1 -> Product/1

== system test_GRM_Airframe/GRM_Airframe/aerodynamics/aerodynamic_via_lookup/calc_derivatives/Cy_derivatives_lookup ==
  aero_pre_lookup : Inport
  Bus Creator1 : BusCreator  Inputs=7
  Bus Selector1 : BusSelector  OutputSignals=k_Mach,f_Mach,k_alB,f_alB,k_beB,f_beB
  Constant : Constant  Value=unc_aero_Cy_scale
  Cy_Interpolation : Interpolation_n-D  NumberOfTableDimensions=3  Table=aero.Cy  ExtrapMethod=Clip  InternalRulePriority=Speed
      settings: InputPortMap=u0,u1,u2,u3,u4,u5
  Cy_delta_l_Interpolation : Interpolation_n-D  NumberOfTableDimensions=3  Table=aero.Cy_delta_l  ExtrapMethod=Clip  InternalRulePriority=Speed
      settings: InputPortMap=u0,u1,u2,u3,u4,u5
  Cy_delta_m_Interpolation : Interpolation_n-D  NumberOfTableDimensions=3  Table=aero.Cy_delta_m  ExtrapMethod=Clip  InternalRulePriority=Speed
      settings: InputPortMap=u0,u1,u2,u3,u4,u5
  Cy_delta_n_Interpolation : Interpolation_n-D  NumberOfTableDimensions=3  Table=aero.Cy_delta_n  ExtrapMethod=Clip  InternalRulePriority=Speed
      settings: InputPortMap=u0,u1,u2,u3,u4,u5
  Cyp_Interpolation : Interpolation_n-D  NumberOfTableDimensions=3  Table=aero.Cyp  ExtrapMethod=Clip  InternalRulePriority=Speed
      settings: InputPortMap=u0,u1,u2,u3,u4,u5
  Cyq_Interpolation : Interpolation_n-D  NumberOfTableDimensions=3  Table=aero.Cyq  ExtrapMethod=Clip  InternalRulePriority=Speed
      settings: InputPortMap=u0,u1,u2,u3,u4,u5
  Cyr_Interpolation : Interpolation_n-D  NumberOfTableDimensions=3  Table=aero.Cyr  ExtrapMethod=Clip  InternalRulePriority=Speed
      settings: InputPortMap=u0,u1,u2,u3,u4,u5
  Product : Product
  Cy_deriv : Outport  VectorParamsAs1DForOutWhenUnconnected=off
  wires:
  Cy_Interpolation/1 -> Product/2  "Cy"
  Cy_delta_n_Interpolation/1 -> Bus Creator1/7  "Cydn"
  Bus Selector1/5 -> Cy_delta_n_Interpolation/5, Cy_delta_m_Interpolation/5, Cy_delta_l_Interpolation/5, Cyr_Interpolation/5, Cyq_Interpolation/5, Cyp_Interpolation/5, Cy_Interpolation/5  "<k_beB>"
  Bus Selector1/6 -> Cy_delta_n_Interpolation/6, Cy_delta_m_Interpolation/6, Cy_delta_l_Interpolation/6, Cyr_Interpolation/6, Cyq_Interpolation/6, Cyp_Interpolation/6, Cy_Interpolation/6  "<f_beB>"
  Bus Selector1/4 -> Cy_delta_n_Interpolation/4, Cy_delta_m_Interpolation/4, Cy_delta_l_Interpolation/4, Cyr_Interpolation/4, Cyq_Interpolation/4, Cyp_Interpolation/4, Cy_Interpolation/4  "<f_alB>"
  Bus Selector1/3 -> Cy_delta_n_Interpolation/3, Cy_delta_m_Interpolation/3, Cy_delta_l_Interpolation/3, Cyr_Interpolation/3, Cyq_Interpolation/3, Cyp_Interpolation/3, Cy_Interpolation/3  "<k_alB>"
  Bus Selector1/1 -> Cy_delta_n_Interpolation/1, Cy_delta_m_Interpolation/1, Cy_delta_l_Interpolation/1, Cyr_Interpolation/1, Cyq_Interpolation/1, Cyp_Interpolation/1, Cy_Interpolation/1  "<k_Mach>"
  Bus Selector1/2 -> Cy_delta_n_Interpolation/2, Cy_delta_m_Interpolation/2, Cy_delta_l_Interpolation/2, Cyr_Interpolation/2, Cyq_Interpolation/2, Cyp_Interpolation/2, Cy_Interpolation/2  "<f_Mach>"
  aero_pre_lookup/1 -> Bus Selector1/1
  Cyp_Interpolation/1 -> Bus Creator1/2  "Cyp"
  Cy_delta_l_Interpolation/1 -> Bus Creator1/5  "Cydl"
  Cy_delta_m_Interpolation/1 -> Bus Creator1/6  "Cydm"
  Bus Creator1/1 -> Cy_deriv/1  "Cy_deriv_bus"
  Cyr_Interpolation/1 -> Bus Creator1/4  "Cyr"
  Cyq_Interpolation/1 -> Bus Creator1/3  "Cyq"
  Constant/1 -> Product/1
  Product/1 -> Bus Creator1/1  "Cy"

== system test_GRM_Airframe/GRM_Airframe/aerodynamics/aerodynamic_via_lookup/calc_derivatives/Cz_derivatives_lookup ==
  aero_pre_lookup : Inport
  Bus Creator1 : BusCreator  Inputs=7
  Bus Selector2 : BusSelector  OutputSignals=k_Mach,f_Mach,k_alB,f_alB,k_beB,f_beB
  Constant : Constant  Value=unc_aero_Cz_scale
  Cz_Interpolation : Interpolation_n-D  NumberOfTableDimensions=3  Table=aero.Cz  ExtrapMethod=Clip  DiagnosticForOutOfRangeInput=Warning  InternalRulePriority=Speed
      settings: InputPortMap=u0,u1,u2,u3,u4,u5
  Cz_delta_l_Interpolation : Interpolation_n-D  NumberOfTableDimensions=3  Table=aero.Cz_delta_l  ExtrapMethod=Clip  DiagnosticForOutOfRangeInput=Warning  InternalRulePriority=Speed
      settings: InputPortMap=u0,u1,u2,u3,u4,u5
  Cz_delta_m_Interpolation : Interpolation_n-D  NumberOfTableDimensions=3  Table=aero.Cz_delta_m  ExtrapMethod=Clip  DiagnosticForOutOfRangeInput=Warning  InternalRulePriority=Speed
      settings: InputPortMap=u0,u1,u2,u3,u4,u5
  Cz_delta_n_Interpolation : Interpolation_n-D  NumberOfTableDimensions=3  Table=aero.Cz_delta_n  ExtrapMethod=Clip  DiagnosticForOutOfRangeInput=Warning  InternalRulePriority=Speed
      settings: InputPortMap=u0,u1,u2,u3,u4,u5
  Czp_Interpolation : Interpolation_n-D  NumberOfTableDimensions=3  Table=aero.Czp  ExtrapMethod=Clip  DiagnosticForOutOfRangeInput=Warning  InternalRulePriority=Speed
      settings: InputPortMap=u0,u1,u2,u3,u4,u5
  Czq_Interpolation : Interpolation_n-D  NumberOfTableDimensions=3  Table=aero.Czq  ExtrapMethod=Clip  DiagnosticForOutOfRangeInput=Warning  InternalRulePriority=Speed
      settings: InputPortMap=u0,u1,u2,u3,u4,u5
  Czr_Interpolation : Interpolation_n-D  NumberOfTableDimensions=3  Table=aero.Czr  ExtrapMethod=Clip  DiagnosticForOutOfRangeInput=Warning  InternalRulePriority=Speed
      settings: InputPortMap=u0,u1,u2,u3,u4,u5
  Product : Product
  Cz_deriv : Outport  VectorParamsAs1DForOutWhenUnconnected=off
  wires:
  Bus Selector2/4 -> Cz_delta_n_Interpolation/4, Cz_delta_m_Interpolation/4, Cz_delta_l_Interpolation/4, Czr_Interpolation/4, Czq_Interpolation/4, Czp_Interpolation/4, Cz_Interpolation/4  "<f_alB>"
  Bus Selector2/2 -> Cz_delta_n_Interpolation/2, Cz_delta_m_Interpolation/2, Cz_delta_l_Interpolation/2, Czr_Interpolation/2, Czq_Interpolation/2, Czp_Interpolation/2, Cz_Interpolation/2  "<f_Mach>"
  Bus Selector2/1 -> Cz_delta_n_Interpolation/1, Cz_delta_m_Interpolation/1, Cz_delta_l_Interpolation/1, Czr_Interpolation/1, Czq_Interpolation/1, Czp_Interpolation/1, Cz_Interpolation/1  "<k_Mach>"
  Bus Selector2/5 -> Cz_delta_n_Interpolation/5, Cz_delta_m_Interpolation/5, Cz_delta_l_Interpolation/5, Czr_Interpolation/5, Czq_Interpolation/5, Czp_Interpolation/5, Cz_Interpolation/5  "<k_beB>"
  Cz_Interpolation/1 -> Product/2  "Cz"
  Cz_delta_m_Interpolation/1 -> Bus Creator1/6  "Czdm"
  Bus Selector2/6 -> Cz_delta_n_Interpolation/6, Cz_delta_m_Interpolation/6, Cz_delta_l_Interpolation/6, Czr_Interpolation/6, Czq_Interpolation/6, Czp_Interpolation/6, Cz_Interpolation/6  "<f_beB>"
  Bus Selector2/3 -> Cz_delta_n_Interpolation/3, Cz_delta_m_Interpolation/3, Cz_delta_l_Interpolation/3, Czr_Interpolation/3, Czq_Interpolation/3, Czp_Interpolation/3, Cz_Interpolation/3  "<k_alB>"
  Cz_delta_n_Interpolation/1 -> Bus Creator1/7  "Czdn"
  Cz_delta_l_Interpolation/1 -> Bus Creator1/5  "Czdl"
  Bus Creator1/1 -> Cz_deriv/1  "Cz_deriv_bus"
  Czq_Interpolation/1 -> Bus Creator1/3  "Czq"
  aero_pre_lookup/1 -> Bus Selector2/1
  Czp_Interpolation/1 -> Bus Creator1/2  "Czp"
  Czr_Interpolation/1 -> Bus Creator1/4  "Czr"
  Constant/1 -> Product/1
  Product/1 -> Bus Creator1/1  "Cz"

== system test_GRM_Airframe/GRM_Airframe/aerodynamics/aerodynamic_via_lookup/calc_derivatives/aerodynamics_pre_lookup ==
  alB : Inport
  beB : Inport  Port=2
  Ma : Inport  Port=3
  Bus Creator1 : BusCreator  Inputs=6
  Prelookup_Mach : PreLookup  BreakpointsData=aero.Ma
  Prelookup_alB : PreLookup  BreakpointsData=aero.alpha
  Prelookup_beB : PreLookup  BreakpointsData=aero.beta
  aero_pre_lookup : Outport  VectorParamsAs1DForOutWhenUnconnected=off
  wires:
  Bus Creator1/1 -> aero_pre_lookup/1  "aero_pre_lookup_bus"
  Prelookup_alB/1 -> Bus Creator1/3  "k_alB"
  Prelookup_alB/2 -> Bus Creator1/4  "f_alB"
  Ma/1 -> Prelookup_Mach/1
  Prelookup_Mach/2 -> Bus Creator1/2  "f_Mach"
  Prelookup_Mach/1 -> Bus Creator1/1  "k_Mach"
  Prelookup_beB/1 -> Bus Creator1/5  "k_beB"
  Prelookup_beB/2 -> Bus Creator1/6  "f_beB"
  alB/1 -> Prelookup_alB/1
  beB/1 -> Prelookup_beB/1
